simulink model "nonlinearsys_nominal"  (R2019b)
settings: Solver=VariableStepAuto  StartTime=0.0  StopTime=10.0  RelTol=1e-3
values from neighbouring files (symbols this model uses):
  g = 9.8    [main_rocketmodel.m]    (also in main_sim_rocket.m; rocket_model.m; sim_lin.m; test_bangbang.m)
  J_T = 40267    [main_rocketmodel.m]    (also in main_sim_rocket.m; rocket_model.m = 10)
  m = 549054    [main_rocketmodel.m]    (also in main_sim_rocket.m; rocket_model.m = 25.4; sim_lin.m; test_bangbang.m)
  t_on = 14.6    [main_rocketmodel.m]    (also in main_sim_rocket.m; test_bangbang.m)
  Ts = 0.001    [main_rocketmodel.m]    (also in main_sim_rocket.m; sim_lin.m; square_sig.m; sum_squares_sig.m)
  x_0 = 0    [main_rocketmodel.m]    (also in main_sim_rocket.m)
  z_0 = 4000    [main_rocketmodel.m]    (also in main_sim_rocket.m; sim_lin.m; test_bangbang.m)
settings Model: Creator=bia  LastModifiedBy=bia
settings DataIOCC: ExternalInput=[t, phi]  LoadExternalInput=on

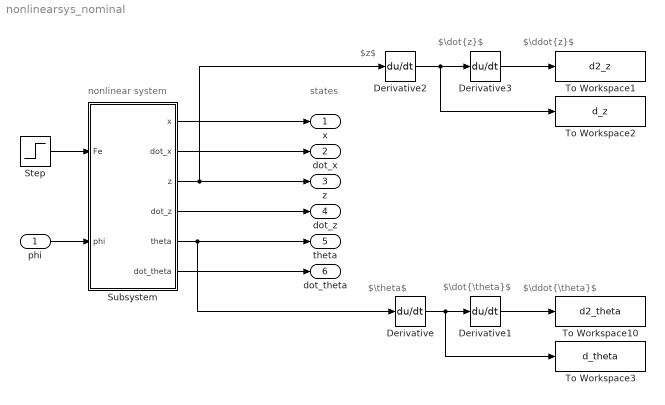
== system nonlinearsys_nominal ==
  note: states
  note: $\theta$
  note: $z$
  note: $\ddot{\theta}$
  note: nonlinear system
  note: $\ddot{z}$
  note: $\dot{z}$
  note: $\dot{\theta}$
  phi : Inport
  Derivative{,1..3} (4 alike) : Derivative
  Step : Step  Time=t_on  Before=0.05*7e6  After=7e6  SampleTime=0
  Subsystem : Subsystem
  To Workspace1 : ToWorkspace  VariableName=d2_z  SampleTime=Ts
  To Workspace10 : ToWorkspace  VariableName=d2_theta  SampleTime=Ts
  To Workspace2 : ToWorkspace  VariableName=d_z  SampleTime=Ts
  To Workspace3 : ToWorkspace  VariableName=d_theta  SampleTime=Ts
  x : Outport
  "dot_x " : Outport  Port=2
  z : Outport  Port=3
  dot_z : Outport  Port=4
  theta : Outport  Port=5
  "dot_theta " : Outport  Port=6
  wires:
  Subsystem/4("dot_z ") -> dot_z/1
  Subsystem/3(z) -> z/1, Derivative2/1
  Derivative2/1 -> To Workspace2/1, Derivative3/1
  Derivative/1 -> Derivative1/1, To Workspace3/1
  Step/1 -> Subsystem/1(Fe)
  Subsystem/6("dot_theta ") -> "dot_theta "/1
  Subsystem/5(theta) -> theta/1, Derivative/1
  Subsystem/2(dot_x) -> "dot_x "/1
  phi/1 -> Subsystem/2(phi)
  Subsystem/1(x) -> x/1
  Derivative3/1 -> To Workspace1/1
  Derivative1/1 -> To Workspace10/1

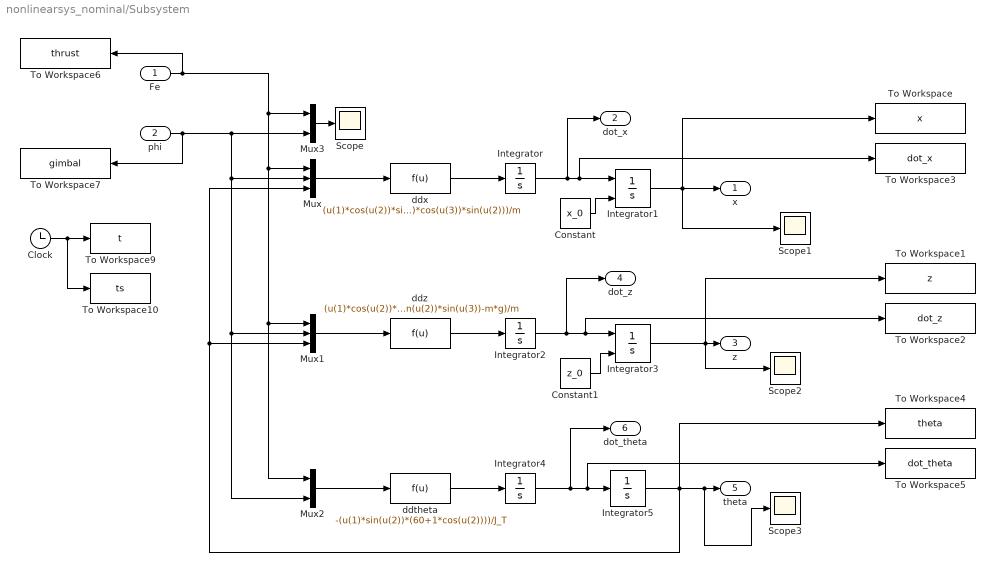
== system nonlinearsys_nominal/Subsystem ==
  Fe : Inport
  phi : Inport  Port=2
  Clock : Clock
  Constant : Constant  Value=x_0  SampleTime=Ts
  Constant1 : Constant  Value=z_0  SampleTime=Ts
  Integrator : Integrator  ContinuousStateAttributes='x_dot'
  Integrator1 : Integrator  InitialConditionSource=external  ContinuousStateAttributes='x'
  Integrator2 : Integrator  ContinuousStateAttributes='z_dot'
  Integrator3 : Integrator  InitialConditionSource=external  InitialCondition=50  LimitOutput=on  LowerSaturationLimit=0  ContinuousStateAttributes='z'
  Integrator4 : Integrator  ContinuousStateAttributes='theta_dot'
  Integrator5 : Integrator
  Mux : Mux  Inputs=3
  Mux1 : Mux  Inputs=3
  Mux2 : Mux  Inputs=2
  Mux3 : Mux  Inputs=2
  Scope{,1..3} (4 alike) : Scope
  To Workspace : ToWorkspace  VariableName=x  SampleTime=Ts
  To Workspace1 : ToWorkspace  VariableName=z  SampleTime=Ts
  To Workspace10 : ToWorkspace  VariableName=ts  SampleTime=Ts
  To Workspace2 : ToWorkspace  VariableName=dot_z  SampleTime=Ts
  To Workspace3 : ToWorkspace  VariableName=dot_x  SampleTime=Ts
  To Workspace4 : ToWorkspace  VariableName=theta  SampleTime=Ts
  To Workspace5 : ToWorkspace  VariableName=dot_theta  SampleTime=Ts
  To Workspace6 : ToWorkspace  VariableName=thrust  SampleTime=Ts
  To Workspace7 : ToWorkspace  VariableName=gimbal  SampleTime=Ts
  To Workspace9 : ToWorkspace  VariableName=t  SampleTime=-1
  ddtheta : Fcn  Expr=-(u(1)*sin(u(2))*(60+1*cos(u(2))))/J_T
  ddx : Fcn  Expr=(u(1)*cos(u(2))*sin(u(3))+u(1)*cos(u(3))*sin(u(2)))/m
  ddz : Fcn  Expr=(u(1)*cos(u(2))*cos(u(3))-u(1)*sin(u(2))*sin(u(3))-m*g)/m
  x : Outport
  dot_x : Outport  Port=2
  z : Outport  Port=3
  "dot_z " : Outport  Port=4
  theta : Outport  Port=5
  "dot_theta " : Outport  Port=6
  wires:
  Integrator1/1 -> Scope1/1, x/1, To Workspace/1
  ddtheta/1 -> Integrator4/1
  Mux/1 -> ddx/1
  ddx/1 -> Integrator/1
  Integrator2/1 -> "dot_z "/1, To Workspace2/1, Integrator3/1
  Mux2/1 -> ddtheta/1
  Fe/1 -> To Workspace6/1, Mux3/1, Mux2/1, Mux1/1, Mux/1
  ddz/1 -> Integrator2/1
  Mux1/1 -> ddz/1
  Integrator/1 -> dot_x/1, To Workspace3/1, Integrator1/1
  phi/1 -> To Workspace7/1, Mux3/2, Mux2/2, Mux1/2, Mux/2
  Integrator3/1 -> To Workspace1/1, Scope2/1, z/1
  Integrator5/1 -> To Workspace4/1, Mux1/3, Mux/3, theta/1, Scope3/1
  Constant1/1 -> Integrator3/2
  Constant/1 -> Integrator1/2
  Integrator4/1 -> "dot_theta "/1, To Workspace5/1, Integrator5/1
  Clock/1 -> To Workspace10/1, To Workspace9/1
  Mux3/1 -> Scope/1
